simulink library "Lib_NM_NewtonRaphsonSolver_EMTAT"  (R2015a)
settings: Solver=ode45  StartTime=0.0  StopTime=10.0  RelTol=1e-3
undefined symbols (not defined in the file): SNR_DX_M, SNR_IC_M, SNR_Mn_M, SNR_Mx_M
Description:
  | Thomas Modules
settings Model: CovSaveCumulativeToWorkspaceVar=on  Creator=jwchapm2  LastModifiedBy=sbianco1
settings OptimizationCC: BlockReduction=off  InlineParams=on  BufferReuse=off  ExpressionDepthLimit=2147483647
settings DebuggingCC: UnderspecifiedInitializationDetection=Classic  MergeDetectMultiDrivingBlocksExec=none  SolverPrmCheckMsg=warning  StateNameClashWarn=warning

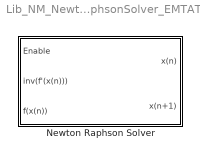
== system Lib_NM_NewtonRaphsonSolver_EMTAT ==
  Newton Raphson Solver : Subsystem  TreatAsAtomicUnit=on  mask(T-MATS: Newton Raphson Solver Library Block){NR_IC_M=SNR_IC_M./abs(SNR_IC_M), NR_dx_Lim_M=SNR_DX_M, NR_Mx_Lim_M=SNR_Mx_M./abs(SNR_IC_M), NR_Mn_Lim_M=SNR_Mn_M./abs(SNR_IC_M), BlkNm_M=double(gcb)}
      mask prompts: NR_IC_M "NR_IC_M - Initial Conditions of Newton Raphson (mx1)"; NR_dx_Lim_M "NR_dx_Lim_M - Newton Raphson step size limit (%) (1x1)"; NR_Mx_Lim_M "NR_Mx_Lim_M - Max limit (1x1 or mx1)"; NR_Mn_Lim_M "NR_Mn_Lim_M - Min Limit (1x1 or mx1)"; BlkNm_M "BlkNm_M - Block Name"
      mask help:
      | Newton Raphson Solver:
      |
      | x(n+1) = x(n) - inverse(f'(x(n)))*f(x(n))
      |
      | Note:
      | inverse(f'(x(n))) is an m x m matrix and f(x(n)) is an m x 1 matrix
      | where m is the length of the initial conditions matrix and number of system independents.
      mask init:
      | if isequal(size(NR_Mx_Lim_M),size(NR_IC_M))
      | elseif isequal(size(NR_Mx_Lim_M),size(1))
      | else
      |     warning('NR_Mx_Lim_M must be the same size as NR_IC_M or a constant')
      | end
      | 
      | if isequal(size(NR_Mn_Lim_M),size(NR_IC_M))
      | elseif isequal(size(NR_Mn_Lim_M),size(1))
      | else
      |     warning('NR_Mn_Lim_M must be the same size as NR_IC_M or a constant')
      | end
      mask Help: web(which('NumMthd_TMATS_NRS.html'),'-helpbrowser')

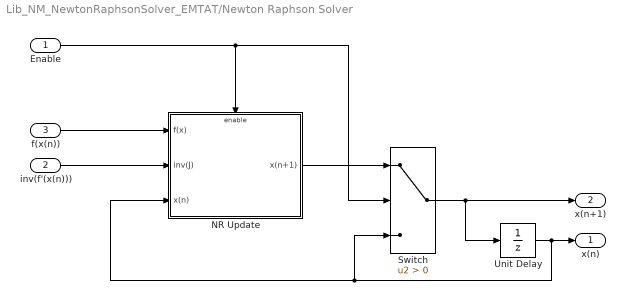
== system Lib_NM_NewtonRaphsonSolver_EMTAT/Newton Raphson Solver ==
  Enable : Inport  PortDimensions=1
  inv(f'(x(n))) : Inport  Port=2  PortDimensions=[length(NR_IC_M),length(NR_IC_M)]
  f(x(n)) : Inport  Port=3  PortDimensions=length(NR_IC_M)
  NR Update : Subsystem
  Switch : Switch  Criteria=u2 > Threshold
  Unit Delay : UnitDelay  InitialCondition=NR_IC_M  SampleTime=-1  HasFrameUpgradeWarning=on
  x(n) : Outport  PortDimensions=length(NR_IC_M)
  x(n+1) : Outport  Port=2  PortDimensions=length(NR_IC_M)
  wires:
  NR Update/1(x(n+1)) -> Switch/1
  inv(f'(x(n)))/1 -> NR Update/2(inv(J))
  f(x(n))/1 -> NR Update/1(f(x))
  Switch/1 -> x(n+1)/1, Unit Delay/1
  Enable/1 -> NR Update/Enable, Switch/2
  Unit Delay/1 -> NR Update/3(x(n)), Switch/3, x(n)/1

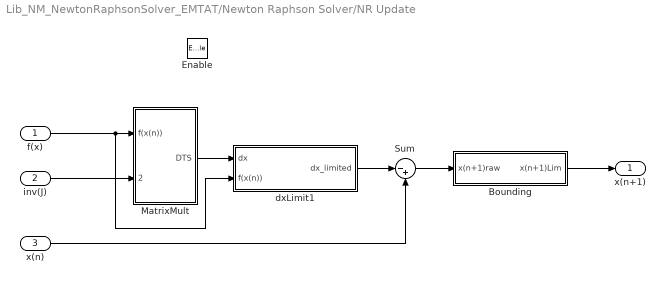
== system Lib_NM_NewtonRaphsonSolver_EMTAT/Newton Raphson Solver/NR Update ==
  f(x) : Inport
  inv(J) : Inport  Port=2
  x(n) : Inport  Port=3
  Enable : EnablePort
  Bounding : Subsystem
  MatrixMult : Subsystem
  Sum : Sum  Inputs=|-+
  dxLimit1 : Subsystem
  x(n+1) : Outport
  wires:
  x(n)/1 -> Sum/2
  Bounding/1(x(n+1)Lim) -> x(n+1)/1
  inv(J)/1 -> MatrixMult/2(inv(f'(x(n))))
  MatrixMult/1(DTS) -> dxLimit1/1(dx)
  Sum/1 -> Bounding/1(x(n+1)raw)
  f(x)/1 -> MatrixMult/1(f(x(n))), dxLimit1/2(f(x(n)))
  dxLimit1/1(dx_limited) -> Sum/1

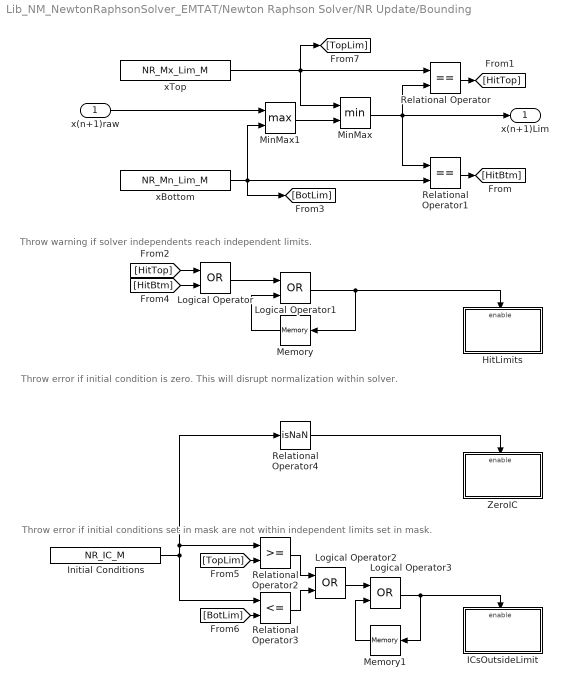
== system Lib_NM_NewtonRaphsonSolver_EMTAT/Newton Raphson Solver/NR Update/Bounding ==
  note: Throw warning if solver independents reach independent limits.
  note: Throw error if initial condition is zero. This will disrupt normalization within solver.
  note: Throw error if initial conditions set in mask are not within independent limits set in mask.
  x(n+1)raw : Inport
  HitLimits : Subsystem
  ICsOutsideLimit : Subsystem
  Initial Conditions : Constant  Value=NR_IC_M
  Logical Operator{,1..3} (4 alike) : Logic  Operator=OR  AllPortsSameDT=off  OutDataTypeStr=boolean
  Memory : Memory  InheritSampleTime=on
  Memory1 : Memory  InheritSampleTime=on
  MinMax : MinMax  Inputs=2
  MinMax1 : MinMax  Function=max  Inputs=2
  Relational Operator : RelationalOperator  Operator===  OutDataTypeStr=boolean
  Relational Operator1 : RelationalOperator  Operator===  OutDataTypeStr=boolean
  Relational Operator2 : RelationalOperator  OutDataTypeStr=boolean
  Relational Operator3 : RelationalOperator  Operator=<=  OutDataTypeStr=boolean
  Relational Operator4 : RelationalOperator  Operator=isNaN  OutDataTypeStr=boolean
  ZeroIC : Subsystem
  xBottom : Constant  Value=NR_Mn_Lim_M
  xTop : Constant  Value=NR_Mx_Lim_M
  x(n+1)Lim : Outport
  wires:
  Relational Operator4/1 -> ZeroIC/Enable
  [BotLim] -> Relational Operator3/2
  Relational Operator2/1 -> Logical Operator2/1
  Memory1/1 -> Logical Operator3/2
  Relational Operator3/1 -> Logical Operator2/2
  Logical Operator2/1 -> Logical Operator3/1
  [TopLim] -> Relational Operator2/2
  Initial Conditions/1 -> Relational Operator3/1, Relational Operator2/1, Relational Operator4/1
  Logical Operator3/1 -> Memory1/1, ICsOutsideLimit/Enable
  Logical Operator1/1 -> Memory/1, HitLimits/Enable
  Memory/1 -> Logical Operator1/2
  [HitBtm] -> Logical Operator/2
  Logical Operator/1 -> Logical Operator1/1
  [HitTop] -> Logical Operator/1
  Relational Operator/1 -> [HitTop]
  Relational Operator1/1 -> [HitBtm]
  MinMax/1 -> x(n+1)Lim/1, Relational Operator/2, Relational Operator1/1
  MinMax1/1 -> MinMax/2
  xTop/1 -> MinMax/1, Relational Operator/1, [TopLim]
  x(n+1)raw/1 -> MinMax1/1
  xBottom/1 -> Relational Operator1/2, MinMax1/2, [BotLim]

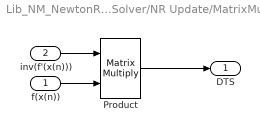
== system Lib_NM_NewtonRaphsonSolver_EMTAT/Newton Raphson Solver/NR Update/MatrixMult ==
  f(x(n)) : Inport
  inv(f'(x(n))) : Inport  Port=2
  Product : Product  Multiplication=Matrix(*)  RndMeth=Zero
  DTS : Outport
  wires:
  inv(f'(x(n)))/1 -> Product/1
  f(x(n))/1 -> Product/2
  Product/1 -> DTS/1

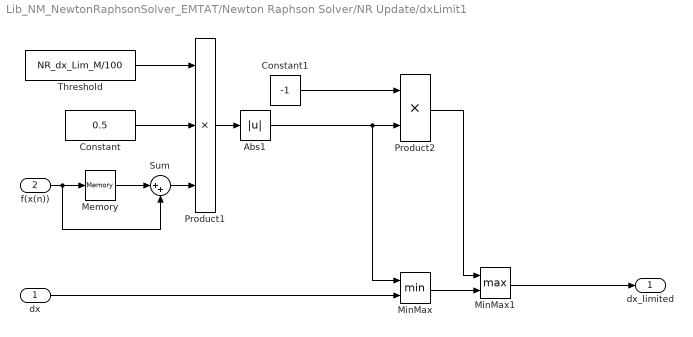
== system Lib_NM_NewtonRaphsonSolver_EMTAT/Newton Raphson Solver/NR Update/dxLimit1 ==
  dx : Inport
  f(x(n)) : Inport  Port=2
  Abs1 : Abs
  Constant : Constant  Value=0.5
  Constant1 : Constant  Value=-1
  Memory : Memory  InheritSampleTime=on
  MinMax : MinMax  Inputs=2
  MinMax1 : MinMax  Function=max  Inputs=2
  Product1 : Product  Inputs=3  RndMeth=Zero
  Product2 : Product  RndMeth=Zero
  Sum : Sum  Inputs=|++
  Threshold : Constant  Value=NR_dx_Lim_M/100
  dx_limited : Outport
  wires:
  MinMax1/1 -> dx_limited/1
  Constant1/1 -> Product2/1
  Product2/1 -> MinMax1/1
  MinMax/1 -> MinMax1/2
  dx/1 -> MinMax/2
  Abs1/1 -> MinMax/1, Product2/2
  Product1/1 -> Abs1/1
  Threshold/1 -> Product1/1
  f(x(n))/1 -> Memory/1, Sum/2
  Constant/1 -> Product1/2
  Memory/1 -> Sum/1
  Sum/1 -> Product1/3

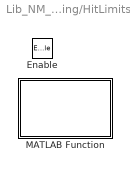
== system Lib_NM_NewtonRaphsonSolver_EMTAT/Newton Raphson Solver/NR Update/Bounding/HitLimits ==
  Enable : EnablePort
  MATLAB Function : MATLAB Function  TreatAsAtomicUnit=on
      settings: PermitHierarchicalResolution=ParametersOnly

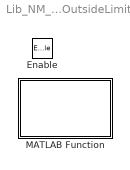
== system Lib_NM_NewtonRaphsonSolver_EMTAT/Newton Raphson Solver/NR Update/Bounding/ICsOutsideLimit ==
  Enable : EnablePort
  MATLAB Function : MATLAB Function  TreatAsAtomicUnit=on
      settings: PermitHierarchicalResolution=ParametersOnly

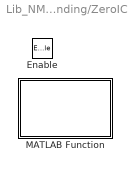
== system Lib_NM_NewtonRaphsonSolver_EMTAT/Newton Raphson Solver/NR Update/Bounding/ZeroIC ==
  Enable : EnablePort
  MATLAB Function : MATLAB Function  TreatAsAtomicUnit=on
      settings: PermitHierarchicalResolution=ParametersOnly

== matlab function Lib_NM_NewtonRaphsonSolver_EMTAT/Newton Raphson Solver/NR Update/Bounding/HitLimits/MATLAB Function ==
  data: BlkNm_M parameter
function fcn(BlkNm_M)
%# Limit Newton Raphson outputs and produce a warning if it occurs
BName = BlkNm_M;
disp(['Warning in ' BName ': Solver limit has been hit, check for system convergence']);

== matlab function Lib_NM_NewtonRaphsonSolver_EMTAT/Newton Raphson Solver/NR Update/Bounding/ICsOutsideLimit/MATLAB Function ==
  data: BlkNm_M parameter
function ICNotInsideLimits(BlkNm_M)
%# Throw error if initial condition is outside bounds on independent.
BName = BlkNm_M;
error(['Error in ' BName ': Initial conditions, SNR_IC_M, of NR Solver are not within the Newton Raphson independent limits, SNR_Mx_M and SNR_Mn_M. Please choose initial condiitons conditions within the prescribed limits.']);

== matlab function Lib_NM_NewtonRaphsonSolver_EMTAT/Newton Raphson Solver/NR Update/Bounding/ZeroIC/MATLAB Function ==
  data: BlkNm_M parameter
function ICIsZero(BlkNm_M)
%# Throw error if initial condition is outside bounds on independent.
BName = BlkNm_M;
error(['Error in ' BName ': Initial conditions, SNR_IC_M, of NR Solver are zero. This will disrupt the normalization within the solver. Please choose non-zero numbers.']);
